simulink model "ANC_Model"  (R2021b)
settings: Solver=FixedStepDiscrete  StartTime=0.0  StopTime=timeout  RelTol=1e-3
undefined symbols (not defined in the file): gain, volume
libraries: dspsnks4 x1, dspvision x1, dspindex x1, dspadpt3 x1
settings Model: Creator=The MathWorks, Inc.  LastModifiedBy=Shera
settings SolverCC: AlgebraicLoopSolver=TrustRegion
settings DataIOCC: ReturnWorkspaceOutputs=off
settings DebuggingCC: SFMachineParentedDataDiag=warning  ArithmeticOperatorsInVariantConditions=warning
settings SFSimCC: CustomCodeUndefinedFunction=UseInterfaceOnly

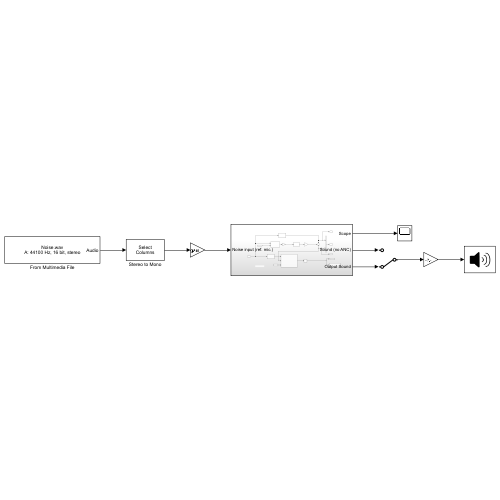
[thumbnail: Simulink's stored preview of the top-level diagram]
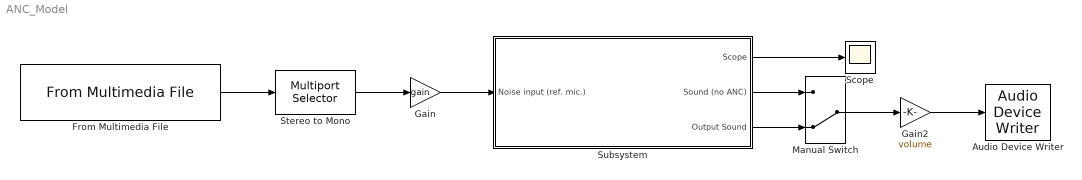
== system ANC_Model ==
  Audio Device Writer : dspsnks4/Audio Device Writer  Driver=DirectSound  Device=Default  InheritSampleRate=on  SampleRate=44100  BitDepth=16-bit integer  BufferSize=4096  NumBuffers=10  DefaultOutputChannelMapping=on  OutputChannelMapping=1:2  OutputNumUnderrunSamples=off  DriverIdx=1  DeviceWarnFlag=''
  From Multimedia File : dspvision/From Multimedia File  inputFilename=Noise.wav  readRange=[1 Inf]  loop=on  numPlays=inf  outputStreams=Audio only  videoDataType=single  audioDataType=double  inheritSampleTime=on  userDefinedSampleTime=1/22050  noAudioOutput=off  isIntensityVideo=off  fourcc=RGB  colorVideoFormat=Separate color signals  outputEOF=off  dataOrg=Column-major  audioFrameSize=1  computeAudioFrameSize=off  outSamplingMode=Sample based
  Gain : Gain  Gain=gain
  Gain2 : Gain  Gain=volume
  Manual Switch : ManualSwitch  CurrentSetting=0
  Scope : Scope
  Stereo to Mono : dspindex/Multiport Selector  rowsOrCols=Columns  idxCellArray=1  idxErrMode=Clip Index
  Subsystem : Subsystem
  wires:
  Manual Switch/1 -> Gain2/1
  Gain2/1 -> Audio Device Writer/1
  Subsystem/1(Scope) -> Scope/1
  Subsystem/2(Sound (no ANC)) -> Manual Switch/1
  Subsystem/3(Output Sound) -> Manual Switch/2
  Stereo to Mono/1 -> Gain/1
  From Multimedia File/1 -> Stereo to Mono/1
  Gain/1 -> Subsystem/1(Noise input (ref. mic.))

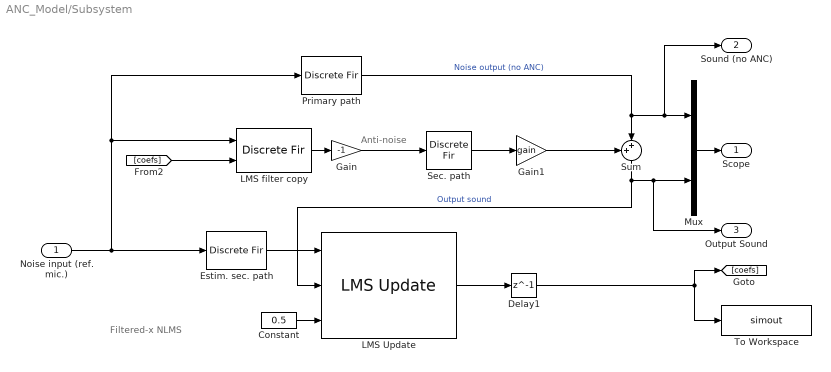
== system ANC_Model/Subsystem ==
  note: Filtered-x NLMS
  note: Anti-noise
  Noise input (ref. mic.) : Inport
  Constant : Constant  Value=0.5
  Delay1 : Delay  DelayLength=1
  Estim. sec. path : DiscreteFir  Coefficients=[0.2 0.02 0.1 -.02 -.03 -0.01]
  Gain : Gain  Gain=-1
  Gain1 : Gain  Gain=gain
  LMS Update : dspadpt3/LMS Update  Method=Normalized LMS  Length=24  StepSizeSource=Input port  StepSize=0.1  LeakageFactor=1.0  InitialConditions=inputweights  EnableAdaptInput=off  EnableResetInput=off  SimulateUsing=Interpreted execution
      settings: SourceProductBaseCode=DS
  LMS filter copy : DiscreteFir  CoefSource=Input port
      settings: InputPortMap=u0,u1
  Mux : Mux  Inputs=2
  Primary path : DiscreteFir  Coefficients=conv([0.02 0.02 0.1 -.02 -.03 -0.01],[.1 -.1 .2 -.2 .3 -.3 .15 -.15])
  Sec. path : DiscreteFir  Coefficients=[0.2 0.02 0.1 -.02 -.03 -0.01]
  Sum : Sum  Inputs=++|
  To Workspace : ToWorkspace  VariableName=simout  SampleTime=-1
      settings: Save2DSignal=2-D array (concatenate along first dimension)
  Scope : Outport
  Sound (no ANC) : Outport  Port=2
  Output Sound : Outport  Port=3
  wires:
  Primary path/1 -> Sound (no ANC)/1, Mux/1, Sum/2  "Noise output (no ANC)"
  Estim. sec. path/1 -> LMS Update/1
  Noise input (ref. mic.)/1 -> Estim. sec. path/1, LMS filter copy/1, Primary path/1
  Constant/1 -> LMS Update/3
  Gain/1 -> Sec. path/1
  LMS filter copy/1 -> Gain/1
  Sum/1 -> LMS Update/2, Output Sound/1, Mux/2  "Output sound"
  Delay1/1 -> To Workspace/1, [coefs]
  Gain1/1 -> Sum/1
  Sec. path/1 -> Gain1/1
  LMS Update/1 -> Delay1/1
  [coefs] -> LMS filter copy/2
  Mux/1 -> Scope/1
